simulink model "RealTimeClock_testt"  (R2023a)
settings: Solver=FixedStepDiscrete  StartTime=0.0  StopTime=10  FixedStep=1e-5  RelTol=1e-3
settings Model: Creator=RT Robotics  LastModifiedBy=RTLab
settings SolverCC: AutoInsertRateTranBlk=on
settings HardwareCC: ProdBitPerLong=64  ProdHWDeviceType=Intel->x86-64 (Linux 64)
settings RTWCC: Description=Simulink Desktop Real-Time  SystemTargetFile=sldrt.tlc  TemplateMakefile=sldrt.tmf  TargetLang=C++  RTWCompilerOptimization=on
settings CodeAppCC: MaxIdLength=95
settings SimulinkDesktopRealTimeCC: TargetLibSuffix=_sldrt.a  TargetPreCompLibLocation=C:\Program Files\MATLAB\R2023a\toolbox\sldrt\lib\win64  TargetLangStandard=C++11 (ISO)

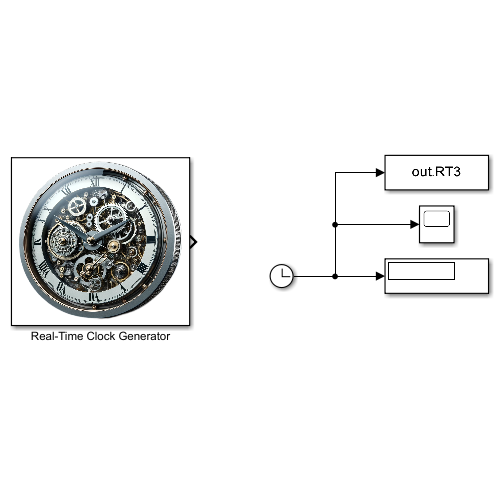
[thumbnail: Simulink's stored preview of the top-level diagram]
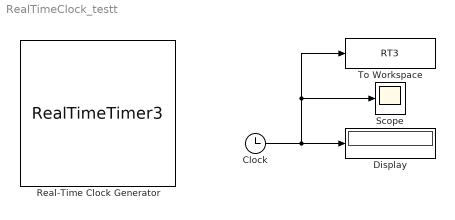
== system RealTimeClock_testt ==
  Clock : Clock
  Display : Display
  Real-Time Clock Generator : S-Function  FunctionName=RealTimeTimer3  Parameters=1e-4  SFunctionDeploymentMode=off  EnableBusSupport=off
      mask Display: image('$imagefile'); % Use "Edit Image" on toolstrip to change.
  Scope : Scope
  To Workspace : ToWorkspace  VariableName=RT3  SaveFormat=Timeseries  SampleTime=-1
  wires:
  Clock/1 -> Scope/1, To Workspace/1, Display/1
